simulink model "serialdecoder1"  (R2018b)
settings: Solver=VariableStepAuto  StartTime=0.0  StopTime=inf  RelTol=1e-3
undefined symbols (not defined in the file or in its folder): serial
libraries: c2000scilib x2, instrumentlib x2
settings Model: Creator=Robert  LastModifiedBy=Robert

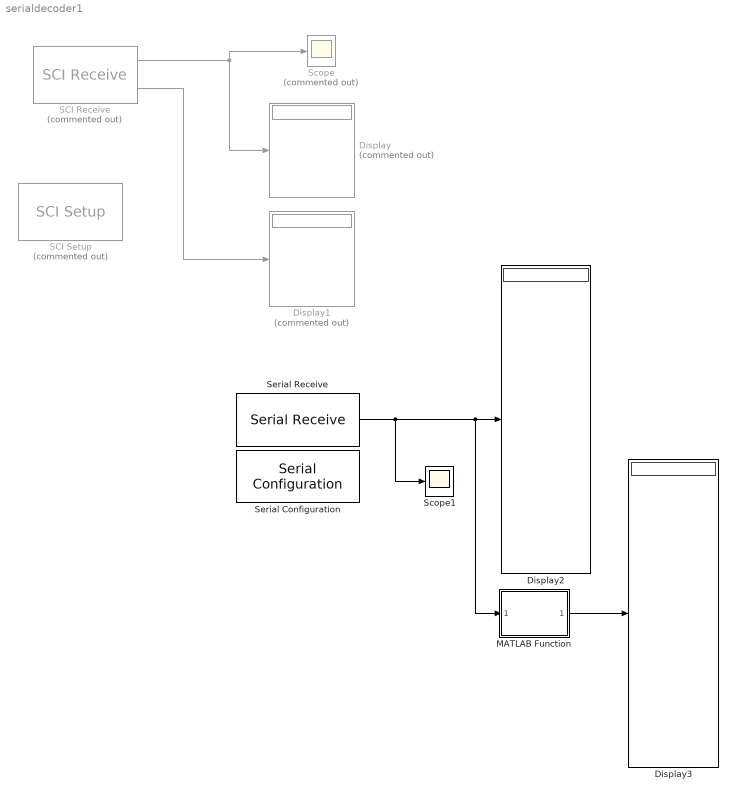
== system serialdecoder1 ==
  Display : Display  Commented=on
  Display1 : Display  Commented=on
  Display2 : Display
  Display3 : Display
  MATLAB Function : MATLAB Function  TreatAsAtomicUnit=on
  SCI Receive : c2000scilib/SCI Receive  Commented=on  module=COM 3  dataHead=65  dataTail=66  dataType=single  dataDim=4  initValue=zeros(1,4)  errOption=Output the last received value  errValue=0  sampleTime=p.Ts  outputStatus=on
      settings: SourceProductName=MATLAB Coder  SourceProductBaseCode=ME
  SCI Setup : c2000scilib/SCI Setup  Priority=-99  Commented=on  commModeA=raw data  baudRateA=115200  charLenA=8  stopBitA=1  parityA=none  timeoutA=1.0  commModeB=raw data  baudRateB=115200  charLenB=8  stopBitB=1  parityB=none  timeoutB=1.0  commModeC=raw data  baudRateC=115200  charLenC=8  stopBitC=1  parityC=none  timeoutC=1.0  commModeD=raw data  baudRateD=115200  charLenD=8  stopBitD=1  parityD=none  timeoutD=1.0
      settings: SourceProductName=MATLAB Coder  SourceProductBaseCode=ME
  Scope : Scope  Commented=on
  Scope1 : Scope
  Serial Configuration : instrumentlib/Serial Configuration  Priority=-200000  ComPortMenu=COM3  ComPort=COM3  ObjConstructor=serial('COM3');  BaudRate=115200  DataBits=8  Parity=none  StopBits=1  FlowControl=none  Timeout=1  ByteOrder=LittleEndian
  Serial Receive : instrumentlib/Serial Receive  ComPortMenu=COM3  ComPort=COM3  ObjConstructor=serial('COM3');  Header=A  Terminator=<none>  DataSize="[1  16]"  DataType=uint8  EnableBlockingMode=on  ActionDataUnavailable=Output custom value  CustomValue=0  SampleTime=0.05
  wires:
  SCI Receive/1 -> Scope/1, Display/1
  SCI Receive/2 -> Display1/1
  Serial Receive/1 -> Scope1/1, MATLAB Function/1(data_u8), Display2/1
  MATLAB Function/1(singles) -> Display3/1

== matlab function serialdecoder1/MATLAB Function ==
  data: data_u8 input; singles output
function singles = bytes2singles(data_u8)

singles = single(zeros(1,4));
singles = typecast(uint8(data_u8),'single');
